simulink model "decode2"  (R2021a)
settings: Solver=VariableStepAuto  StartTime=0.0  StopTime=10.0  RelTol=1e-3
libraries: dsp_blocks x6
settings Model: Creator=nathanalemayehu  LastModifiedBy=nathanalemayehu

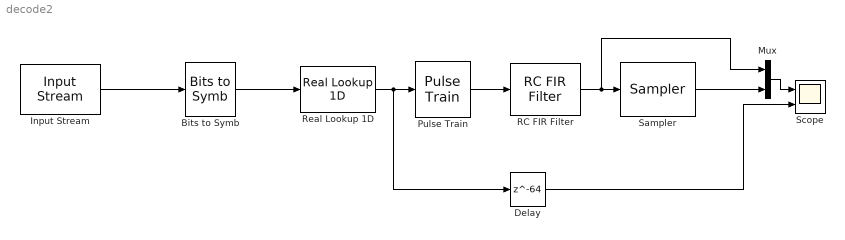
== system decode2 ==
  Bits to Symb : dsp_blocks/Conversions/Bits to Symb
  Delay : Delay  DelayLength=64
  Input Stream : dsp_blocks/Sources//Sinks/Input Stream  period=10  width=1  fname=rand.mat
  Mux : Mux  Inputs=2
  Pulse Train : dsp_blocks/Conversions/Pulse Train  period=10
  RC FIR Filter : dsp_blocks/Filters/RC FIR Filter  period=10  beta=0.5  root=off  filt_len=128  win_type=on
  Real Lookup 1D : dsp_blocks/Conversions/Real Lookup 1D  table=[-1 1]
  Sampler : dsp_blocks/Conversions/Sampler  offset=64  samp_period=10
  Scope : Scope  NumInputPorts=2
  wires:
  Input Stream/1 -> Bits to Symb/1
  Sampler/1 -> Mux/2
  Delay/1 -> Scope/2
  Mux/1 -> Scope/1
  RC FIR Filter/1 -> Mux/1, Sampler/1
  Bits to Symb/1 -> Real Lookup 1D/1
  Pulse Train/1 -> RC FIR Filter/1
  Real Lookup 1D/1 -> Delay/1, Pulse Train/1
